simulink model "notLinModel_S"  (R2021b)
settings: Solver=ode45  StartTime=0.0  StopTime=1  MaxStep=0.0005  RelTol=1e-8
values from neighbouring files (symbols this model uses):
  c = 0.2557    [Dynamic_model_lin.m]    (also in Dynamic_model_not_lin.m = 0.179; Dynamic_model_not_lin_filt.m)
  C_magnetic = 3.73e-6    (= 3.73e-06)    [Dynamic_model_lin.m]    (also in Dynamic_model_not_lin.m; Dynamic_model_not_lin_filt.m)
  gap = 3E-4    (= 0.0003)    [Dynamic_model_lin.m]    (also in Dynamic_model_not_lin.m; Dynamic_model_not_lin_filt.m)
  k = 1272.8    [Dynamic_model_lin.m]    (also in Dynamic_model_not_lin.m = 309.2904; Dynamic_model_not_lin_filt.m)
  mass = 0.48    [Dynamic_model_lin.m]    (also in Dynamic_model_not_lin.m = 0.18; Dynamic_model_not_lin_filt.m)
libraries: simulink x1
settings Model: Creator=danli  LastModifiedBy=danli
settings SolverCC: AlgebraicLoopSolver=TrustRegion
settings DebuggingCC: SFMachineParentedDataDiag=warning

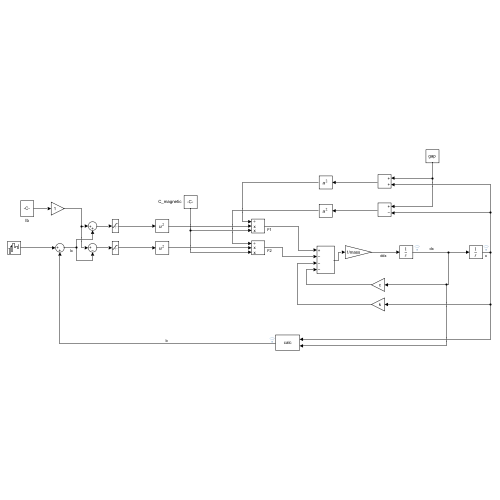
[thumbnail: Simulink's stored preview of the top-level diagram]
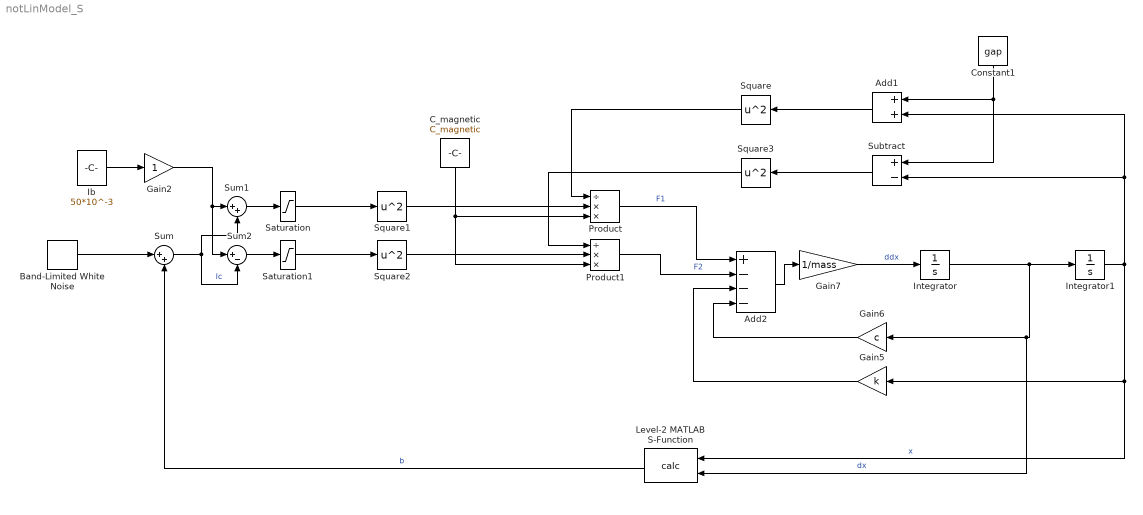
== system notLinModel_S ==
  Add1 : Sum
  Add2 : Sum  Inputs=+---
  Band-Limited White Noise : simulink/Sources/Band-Limited White Noise  Cov=[0.0000000003]  Ts=0.0001  seed=[23341]
  C_magnetic : Constant  Value=C_magnetic
  Constant1 : Constant  Value=gap
  Gain2 : Gain
  Gain5 : Gain  Gain=k
  Gain6 : Gain  Gain=c
  Gain7 : Gain  Gain=1/mass
  Ib : Constant  Value=50*10^-3
  Integrator : Integrator
  Integrator1 : Integrator  InitialCondition=50*10^-6
  Level-2 MATLAB S-Function : M-S-Function  FunctionName=calc
  Product : Product  Inputs=/**
  Product1 : Product  Inputs=/**
  Saturation : Saturate  UpperLimit=2  LowerLimit=0
  Saturation1 : Saturate  UpperLimit=2  LowerLimit=0
  Square{,1..3} (4 alike) : Math  Operator=square  SaturateOnIntegerOverflow=on
  Subtract : Sum  Inputs=+-
  Sum : Sum  Inputs=|++
  Sum1 : Sum  Inputs=|++
  Sum2 : Sum  Inputs=|+-
  wires:
  Ib/1 -> Gain2/1
  Sum1/1 -> Saturation/1
  Sum2/1 -> Saturation1/1
  Sum/1 -> Sum1/2, Sum2/2  "Ic"
  Gain2/1 -> Sum2/1, Sum1/1
  Integrator1/1 -> Add1/2, Subtract/2, Level-2 MATLAB S-Function/1, Gain5/1  "x"
  Saturation1/1 -> Square2/1
  Saturation/1 -> Square1/1
  Square2/1 -> Product1/2
  Constant1/1 -> Subtract/1, Add1/1
  Square1/1 -> Product/2
  Gain6/1 -> Add2/4
  Integrator/1 -> Level-2 MATLAB S-Function/2, Gain6/1, Integrator1/1  "dx"
  Gain5/1 -> Add2/3
  Product1/1 -> Add2/2  "F2"
  Subtract/1 -> Square3/1
  Square/1 -> Product/1
  Add1/1 -> Square/1
  Add2/1 -> Gain7/1
  Product/1 -> Add2/1  "F1"
  Square3/1 -> Product1/1
  C_magnetic/1 -> Product/3, Product1/3
  Gain7/1 -> Integrator/1  "ddx"
  Band-Limited White Noise/1 -> Sum/1
  Level-2 MATLAB S-Function/1 -> Sum/2  "b"
